simulink model "Stabilize_HIL"  (R2017b)
settings: Solver=FixedStepDiscrete  StartTime=0.0  StopTime=10.0  RelTol=1e-3
undefined symbols (not defined in the file): DEG2RAD, DiscIntNeverNeededParam, Kd_PITCH_AngleRate, Kd_ROLL_AngleRate, Kd_YAW_AngleRate, Ki_PITCH_AngleRate, Ki_ROLL_AngleRate, Ki_YAW_AngleRate, Kp_PITCH_ANGLE, Kp_PITCH_AngleRate, Kp_ROLL_ANGLE, Kp_ROLL_AngleRate, Kp_YAW_AngleRate, Kpxp, Kpyp, Kpzp, Kvxd, Kvxi, Kvxp, Kvyd, Kvyi, Kvyp, Kvzd, Kvzi, Kvzp, MAX_CONTROL_ANGLE_PITCH, MAX_CONTROL_ANGLE_RATE_PITCH, MAX_CONTROL_ANGLE_RATE_ROLL, MAX_CONTROL_ANGLE_RATE_Y, MAX_CONTROL_ANGLE_ROLL, MAX_CONTROL_VELOCITY_XY, MAX_CONTROL_VELOCITY_Z, RGBLED_COLOR_ENUM, RGBLED_MODE_ENUM, Saturation_I_ah, Saturation_I_az, Saturation_I_RP_Max, Saturation_I_RP_Min, Saturation_I_Y_Max, Saturation_I_Y_Min, THR_HOVER
libraries: simulink x7, pixhawk_slib_sensors_actuators x4, pixhawk_slib_uORB_RW x2
settings Model: Creator=wsh  LastModifiedBy=Mr Wang
settings OptimizationCC: DefaultParameterBehavior=Inlined  MaxStackSize=64
settings DebuggingCC: ParameterTunabilityLossMsg=error
settings HardwareCC: ProdBitPerPointer=32  ProdBitPerSizeT=32  ProdBitPerPtrDiffT=32  ProdLargestAtomicInteger=Long  ProdLargestAtomicFloat=Double  ProdWordSize=32  ProdHWDeviceType=ARM Compatible->ARM Cortex
settings SFSimCC: MATLABDynamicMemAlloc=off
settings RTWCC: SystemTargetFile=ert.tlc  HardwareBoard=Pixhawk PX4  TemplateMakefile=ert_default_tmf  GenerateReport=on  Toolchain=Pixhawk Toolchain  IncludeHyperlinkInReport=on  LaunchReport=on  GenerateTraceInfo=on  GenerateTraceReport=on  GenerateTraceReportSl=on  GenerateTraceReportSf=on  GenerateTraceReportEml=on
settings CodeAppCC: ForceParamTrailComments=on  IgnoreCustomStorageClasses=off  OperatorAnnotations=on  SimulinkDataObjDesc=on  SFDataObjDesc=on  MATLABFcnDesc=on  InsertBlockDesc=on  StateflowObjectComments=on  MATLABSourceComments=on
settings ERTTargetCC: MultiwordLength=2048  ERTCustomFileTemplate=PX4_codertarget_file_process.tlc

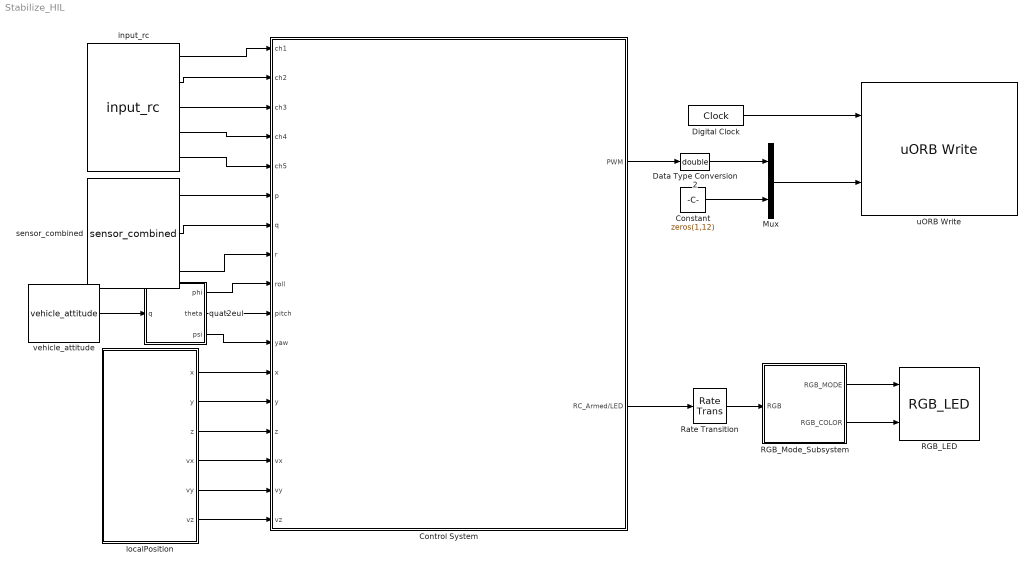
== system Stabilize_HIL ==
  Constant : Constant  Value=zeros(1,12)
  Control System : Subsystem
      mask Display: image('icon\pixhawk.png');
  Data Type Conversion2 : DataTypeConversion  OutDataTypeStr=double
  Digital Clock : DigitalClock  SampleTime=-1
  Mux : Mux  Inputs=2
  RGB_LED : pixhawk_slib_sensors_actuators/RGB_LED
      settings: SourceProductName=Pixhawk Target Blocks
  RGB_Mode_Subsystem : Subsystem
  Rate Transition : RateTransition  OutPortSampleTime=1
  input_rc : pixhawk_slib_sensors_actuators/input_rc  Description=|  sampletime=0.004  channel1=on  channel2=on  channel3=on  channel4=on  channel5=on  channel6=off  channel7=off  channel8=off  channel9=off  channel10=off  channel11=off  channel12=off  channel13=off  channel14=off  channel15=off  channel16=off  channel17=off  channel18=off  ch_count=off  rssi=off  rc_failsafe=off  rc_lost=off  rc_inputsource=off
      | RC Input Block
      | 
      | This block provides user input control to the model.
      | It uses the input_rc uORB topic.
      | 
      | The user has the ability to choose which channels are available as outputs from this block and also some optional outputs. These include 
      | Channels 1 through 18
      | double data type indicating the PWM value from the controller 
      | measured pulse widths for each of the supported channels 
      | Channel Count 
      | uint32 data type of the number of channels which are detector by the PX4 
      | RC Failsafe 
      | boolean data types indicating that the RC Tx is sending the FailSafe signal (if equipped and properly setup) 
      | explicit failsafe flag: true on TX failure or TX out of range , false otherwise. 
      | Only the true state is reliable, as there are some (PPM) receivers on the market going into failsafe without telling us explicitly. 
      | RC Input Source 
      | Enumeration data type indicating which source the RC input is from. 
      | Valid values are found in the ENUM file: RC_INPUT_SOURCE_ENUM.m 
      |           Enumeration members for class 'RC_INPUT_SOURCE_ENUM':
      |           RCINPUT_SOURCE_UNKNOWN         (0)
      |           RCINPUT_SOURCE_PX4FMU_PPM      (1)
      |           RCINPUT_SOURCE_PX4IO_PPM       (2)
      |           RCINPUT_SOURCE_PX4IO_SPEKTRUM  (3)
      |           RCINPUT_SOURCE_PX4IO_SBUS      (4)
      |           RCINPUT_SOURCE_PX4IO_ST24      (5)
      |           RCINPUT_SOURCE_MAVLINK         (6)
      |           RCINPUT_SOURCE_QURT            (7)
      |           RCINPUT_SOURCE_PX4FMU_SPEKTRUM (8)
      |           RCINPUT_SOURCE_PX4FMU_SBUS     (9)
      |           RCINPUT_SOURCE_PX4FMU_ST24     (10)
      |           RCINPUT_SOURCE_PX4FMU_SUMD     (11)
      |           RCINPUT_SOURCE_PX4FMU_DSM      (12)
      |           RCINPUT_SOURCE_PX4IO_SUMD      (13)
      | 
      | RSSI - Receive signal strength index 
      | receive signal strength indicator (RSSI): < 0: Undefined, 0: no signal, 255: full reception 
      | RC Lost Connection 
      | boolean data type indicating RC receiver connection status 
      | True, if no frame has arrived in the expected time, false otherwise. 
      | True usally means that the receiver has been disconnected, but can also indicate a radio link loss on "stupid" systems. 
      | Will remain false, if a RX with failsafe option continues to transmit frames after a link loss. 
      |   
      | Sample Model: px4demo_input_rc.slx
      settings: SourceProductName=Pixhawk Target Blocks
  "localPosition " : Subsystem
  quat2eul : MATLAB Function  TreatAsAtomicUnit=on
  sensor_combined : pixhawk_slib_sensors_actuators/sensor_combined  Description=|  sampletime=0.004  show_mag=off  show_acc=off  show_gyro=on  show_baro=off  show_ts=off
      | Sensor Combined Block
      | 
      | This block enables access to the various sensors available on the px4fmu-v2 hardware.  
      | The user can use these signals in the Simulink control model.  
      | The sample time needs to be provided in the mask dialog.  
      | Optional output ports can also be selected.  
      | Refer to the sample model: px4demo_attitude_control.slx
      | 
      | Signal definitions: 
      | Magnetometer (x,y,z) - single values – Magnetic field in NED body frame, in Gauss 
      | Accelerometer (x,y,z) - single values – Acceleration in NED body frame, in m/s^2 
      | Gyroscope (p,q,r) - single values – Angular velocity in radians per second 
      | Barometer (Altitude) - single value – Barometric pressure, already temperature compensated (millibars) 
      | RunTime (timestamp) - double value – Timestamp in microseconds since boot, from gyro 
      |   
      | The sensor_combined block needs to have the px4io service running on the PX4 hardware in order to get valid signal values.
      settings: SourceProductName=Pixhawk Target Blocks
  uORB Write : pixhawk_slib_uORB_RW/uORB Write  uORB_Topic_str='actuator_outputs'  BlockOutputCount=2  OutputBoolean_1=on  uORB_Param_Name1='timestamp'  uORB_Param_Name_DT1=double  VectorScalar_1=1  OutputBoolean_2=on  uORB_Param_Name2='output'  uORB_Param_Name_DT2=double  VectorScalar_2=16  OutputBoolean_3=off  uORB_Param_Name3='timestamp_time'  uORB_Param_Name_DT3=double  VectorScalar_3=1  OutputBoolean_4=off  uORB_Param_Name4='gyro_temp'  uORB_Param_Name_DT4=single  VectorScalar_4=3  OutputBoolean_5=off  uORB_Param_Name5='vel_ned_valid'  uORB_Param_Name_DT5=boolean  VectorScalar_5=1  Ts=-1  MsgSizeOf=0
      settings: SourceProductName=Pixhawk Target Blocks
  vehicle_attitude : pixhawk_slib_sensors_actuators/vehicle_attitude  Description=|  sampletime=0.004  show_r=off  show_p=off  show_y=off  show_q=on  show_ts=off
      | This block gives access to the running service that calculates the vehicle’s attitude.  A uORB topic (vehicle_attitude (attitude measurements)) publisher MUST be running in order for this block to provide valid signal values.  The available ones as of v1.3 are: 
      | attitude_estimator_ekf – EKF-Extended Kalman Filter for attitude estimation 
      | attitude_estimator_so3 – SO(3)-attitude estimation by using accelerometer, gyroscopes and magnetometer 
      | One of these MUST be running on the px4fmu in order for this block to return valid values.  Refer to the sample model: px4demo_attitude_control.slx. Attitude in NED (North-East-Down) body frame in SI units. 
      | Signal definitions: 
      | Roll – single value, Roll angle (rad, Tait-Bryan, NED) 
      | Pitch – single value, Pitch angle (rad, Tait-Bryan, NED) 
      | Yaw – single value, Yaw angle (rad, Tait-Bryan, NED) 
      | Quaternion (NED) – single(4) values (optional based on the uORB publisher)
      settings: SourceProductName=Pixhawk Target Blocks
  wires:
  sensor_combined/1 -> Control System/6(p)
  sensor_combined/3 -> Control System/8(r)
  sensor_combined/2 -> Control System/7(q)
  input_rc/5 -> Control System/5(ch5)
  input_rc/4 -> Control System/4(ch4)
  input_rc/3 -> Control System/3(ch3)
  input_rc/2 -> Control System/2(ch2)
  input_rc/1 -> Control System/1(ch1)
  quat2eul/3(psi) -> Control System/11(yaw)
  quat2eul/1(phi) -> Control System/9(roll)
  "localPosition "/6(vz) -> Control System/17(vz)
  "localPosition "/1(x) -> Control System/12(x)
  "localPosition "/3(z) -> Control System/14(z)
  "localPosition "/4(vx) -> Control System/15(vx)
  "localPosition "/2(y) -> Control System/13(y)
  vehicle_attitude/1 -> quat2eul/1(q)
  "localPosition "/5(vy) -> Control System/16(vy)
  quat2eul/2(theta) -> Control System/10(pitch)
  Control System/2(RC_Armed/LED) -> Rate Transition/1
  RGB_Mode_Subsystem/1(RGB_MODE) -> RGB_LED/1
  RGB_Mode_Subsystem/2(RGB_COLOR) -> RGB_LED/2
  Data Type Conversion2/1 -> Mux/1
  Control System/1(PWM) -> Data Type Conversion2/1
  Rate Transition/1 -> RGB_Mode_Subsystem/1(RGB)
  Constant/1 -> Mux/2
  Digital Clock/1 -> uORB Write/1
  Mux/1 -> uORB Write/2

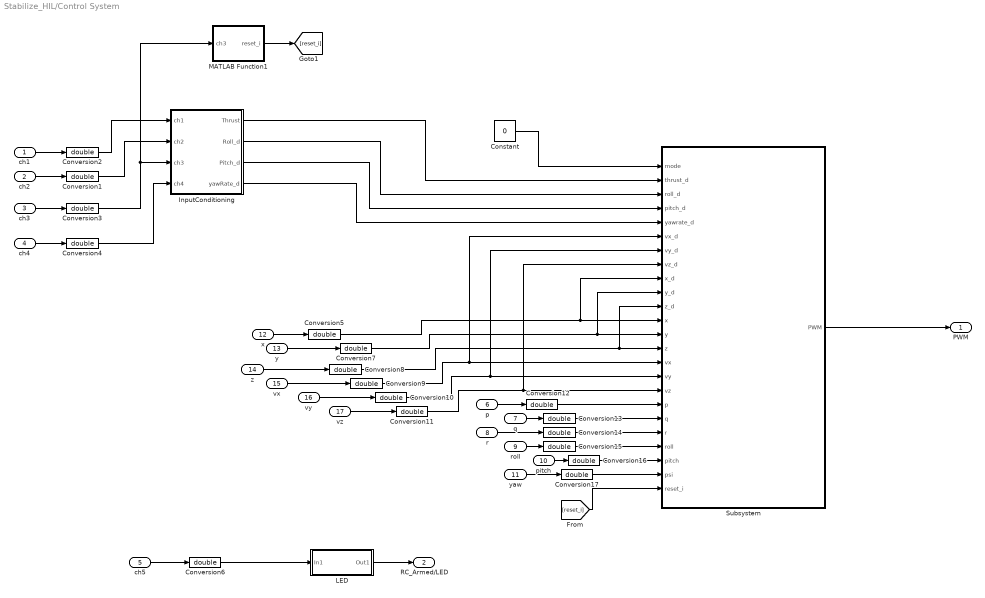
== system Stabilize_HIL/Control System ==
  ch1 : Inport  OutDataTypeStr=uint16  PortDimensions=1
  ch2 : Inport  Port=2  OutDataTypeStr=uint16  PortDimensions=1
  ch3 : Inport  Port=3  OutDataTypeStr=uint16  PortDimensions=1
  ch4 : Inport  Port=4  OutDataTypeStr=uint16  PortDimensions=1
  ch5 : Inport  Port=5  OutDataTypeStr=uint16  PortDimensions=1  Interpolate=off
  p : Inport  Port=6  PortDimensions=1
  q : Inport  Port=7  PortDimensions=1
  r : Inport  Port=8  PortDimensions=1
  roll : Inport  Port=9  PortDimensions=1
  pitch : Inport  Port=10  PortDimensions=1
  yaw : Inport  Port=11  PortDimensions=1
  x : Inport  Port=12
  y : Inport  Port=13
  z : Inport  Port=14
  vx : Inport  Port=15
  vy : Inport  Port=16
  vz : Inport  Port=17
  Constant : Constant  Value=0
  Conversion{1..17} (17 alike) : DataTypeConversion  OutDataTypeStr=double
  InputConditioning : Subsystem
  "LED " : Subsystem
  MATLAB Function1 : MATLAB Function  TreatAsAtomicUnit=on
  Subsystem : Subsystem
  PWM : Outport
  RC_Armed/LED : Outport  Port=2  PortDimensions=1
  wires:
  ch3/1 -> Conversion3/1
  ch5/1 -> Conversion6/1
  ch4/1 -> Conversion4/1
  Conversion4/1 -> InputConditioning/4(ch4)
  ch1/1 -> Conversion2/1
  ch2/1 -> Conversion1/1
  Conversion1/1 -> InputConditioning/2(ch2)
  x/1 -> Conversion5/1
  y/1 -> Conversion7/1
  z/1 -> Conversion8/1
  Constant/1 -> Subsystem/1(mode)
  roll/1 -> Conversion15/1
  pitch/1 -> Conversion16/1
  p/1 -> Conversion12/1
  q/1 -> Conversion13/1
  r/1 -> Conversion14/1
  yaw/1 -> Conversion17/1
  vz/1 -> Conversion11/1
  vy/1 -> Conversion10/1
  vx/1 -> Conversion9/1
  InputConditioning/2(Roll_d) -> Subsystem/3(roll_d)
  InputConditioning/3(Pitch_d) -> Subsystem/4(pitch_d)
  InputConditioning/1(Thrust) -> Subsystem/2(thrust_d)
  InputConditioning/4(yawRate_d) -> Subsystem/5(yawrate_d)
  Conversion5/1 -> Subsystem/12(x), Subsystem/9(x_d)
  Conversion7/1 -> Subsystem/13(y), Subsystem/10(y_d)
  Conversion8/1 -> Subsystem/14(z), Subsystem/11(z_d)
  Conversion9/1 -> Subsystem/15(vx), Subsystem/6(vx_d)
  Conversion10/1 -> Subsystem/16(vy), Subsystem/7(vy_d)
  Conversion11/1 -> Subsystem/17(vz), Subsystem/8(vz_d)
  Conversion12/1 -> Subsystem/18(p)
  Conversion13/1 -> Subsystem/19(q)
  Conversion14/1 -> Subsystem/20(r)
  Conversion15/1 -> Subsystem/21(roll)
  Conversion16/1 -> Subsystem/22(pitch)
  Conversion17/1 -> Subsystem/23(psi)
  Conversion3/1 -> MATLAB Function1/1(ch3), InputConditioning/3(ch3)
  MATLAB Function1/1(reset_i) -> [reset_i]
  [reset_i] -> Subsystem/24(reset_i)
  Conversion2/1 -> InputConditioning/1("ch1 ")
  Subsystem/1(PWM) -> PWM/1
  Conversion6/1 -> "LED "/1(In1)
  "LED "/1(Out1) -> RC_Armed/LED/1

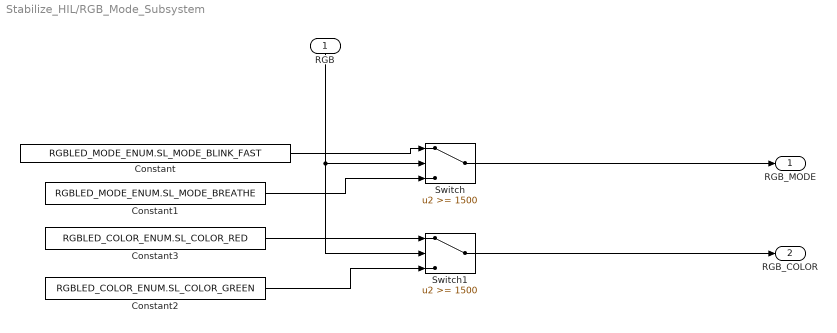
== system Stabilize_HIL/RGB_Mode_Subsystem ==
  RGB : Inport
  Constant : Constant  Value=RGBLED_MODE_ENUM.SL_MODE_BLINK_FAST  OutDataTypeStr=Enum: RGBLED_MODE_ENUM
  Constant1 : Constant  Value=RGBLED_MODE_ENUM.SL_MODE_BREATHE  OutDataTypeStr=Enum: RGBLED_MODE_ENUM
  Constant2 : Constant  Value=RGBLED_COLOR_ENUM.SL_COLOR_GREEN  OutDataTypeStr=Enum: RGBLED_COLOR_ENUM
  Constant3 : Constant  Value=RGBLED_COLOR_ENUM.SL_COLOR_RED  OutDataTypeStr=Enum: RGBLED_COLOR_ENUM
  Switch : Switch  Threshold=1500
  Switch1 : Switch  Threshold=1500
  RGB_MODE : Outport
  RGB_COLOR : Outport  Port=2
  wires:
  RGB/1 -> Switch1/2, Switch/2
  Constant/1 -> Switch/1
  Constant1/1 -> Switch/3
  Switch/1 -> RGB_MODE/1
  Constant3/1 -> Switch1/1
  Constant2/1 -> Switch1/3
  Switch1/1 -> RGB_COLOR/1

== system Stabilize_HIL/localPosition  ==
  Bus Selector2 : BusSelector  OutputSignals=x,y,z,vx,vy,vz
  uORB Read Function-Call Trigger : pixhawk_slib_uORB_RW/uORB Read Function-Call Trigger  uORB_Topic_str='vehicle_local_position'  BusObjVar=Bus: vehicle_local_position_SL  uORB_Interval=1  AsyncOutput=off  Fcn_call_select=Generate Function Call Signal  TaskName='Task1'  Poll_timeout=100  Ts=-1
      settings: SourceProductName=Pixhawk Target Blocks
  x : Outport
  y : Outport  Port=2
  z : Outport  Port=3
  vx : Outport  Port=4
  vy : Outport  Port=5
  vz : Outport  Port=6
  wires:
  uORB Read Function-Call Trigger/1 -> Bus Selector2/1
  Bus Selector2/6 -> vz/1  "<vz>"
  Bus Selector2/5 -> vy/1  "<vy>"
  Bus Selector2/4 -> vx/1  "<vx>"
  Bus Selector2/1 -> x/1  "<x>"
  Bus Selector2/2 -> y/1  "<y>"
  Bus Selector2/3 -> z/1  "<z>"

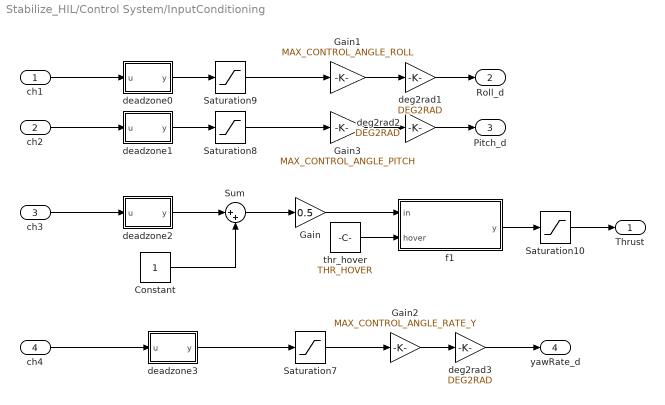
== system Stabilize_HIL/Control System/InputConditioning ==
  "ch1 " : Inport
  ch2 : Inport  Port=2
  ch3 : Inport  Port=3
  ch4 : Inport  Port=4
  Constant : Constant
  Gain : Gain  Gain=0.5
  Gain1 : Gain  Gain=MAX_CONTROL_ANGLE_ROLL  OutDataTypeStr=Inherit: Inherit via back propagation
  Gain2 : Gain  Gain=MAX_CONTROL_ANGLE_RATE_Y
  Gain3 : Gain  Gain=MAX_CONTROL_ANGLE_PITCH  OutDataTypeStr=Inherit: Inherit via back propagation
  Saturation10 : Saturate  UpperLimit=1  LowerLimit=0
  Saturation7 : Saturate  UpperLimit=1  LowerLimit=-1
  Saturation8 : Saturate  UpperLimit=1  LowerLimit=-1
  Saturation9 : Saturate  UpperLimit=1  LowerLimit=-1
  Sum : Sum  Inputs=|++
  deadzone0 : MATLAB Function  TreatAsAtomicUnit=on
  deadzone1 : MATLAB Function  TreatAsAtomicUnit=on
  deadzone2 : MATLAB Function  TreatAsAtomicUnit=on
  deadzone3 : MATLAB Function  TreatAsAtomicUnit=on
  deg2rad1 : Gain  Gain=DEG2RAD
  deg2rad2 : Gain  Gain=DEG2RAD
  deg2rad3 : Gain  Gain=DEG2RAD
  f1 : MATLAB Function  TreatAsAtomicUnit=on
  "thr_hover " : Constant  Value=THR_HOVER
  Thrust : Outport
  Roll_d : Outport  Port=2
  Pitch_d : Outport  Port=3
  yawRate_d : Outport  Port=4
  wires:
  deadzone2/1(y) -> Sum/1
  ch3/1 -> deadzone2/1(u)
  deadzone1/1(y) -> Saturation8/1
  Saturation10/1 -> Thrust/1
  deadzone0/1(y) -> Saturation9/1
  "ch1 "/1 -> deadzone0/1(u)
  ch2/1 -> deadzone1/1(u)
  Saturation9/1 -> Gain1/1
  Saturation8/1 -> Gain3/1
  Gain3/1 -> deg2rad2/1
  Constant/1 -> Sum/2
  Sum/1 -> Gain/1
  Gain1/1 -> deg2rad1/1
  deg2rad1/1 -> Roll_d/1
  deg2rad2/1 -> Pitch_d/1
  Saturation7/1 -> Gain2/1
  deadzone3/1(y) -> Saturation7/1
  ch4/1 -> deadzone3/1(u)
  Gain2/1 -> deg2rad3/1
  deg2rad3/1 -> yawRate_d/1
  "thr_hover "/1 -> f1/2(hover)
  Gain/1 -> f1/1(in)
  f1/1(y) -> Saturation10/1

== system Stabilize_HIL/Control System/LED  ==
  In1 : Inport
  Compare To Constant3 : simulink/Logic and Bit Operations/Compare To Constant  relop=>=  const=uint16(1500)  OutDataTypeStr=boolean
  Out1 : Outport
  wires:
  Compare To Constant3/1 -> Out1/1
  In1/1 -> Compare To Constant3/1

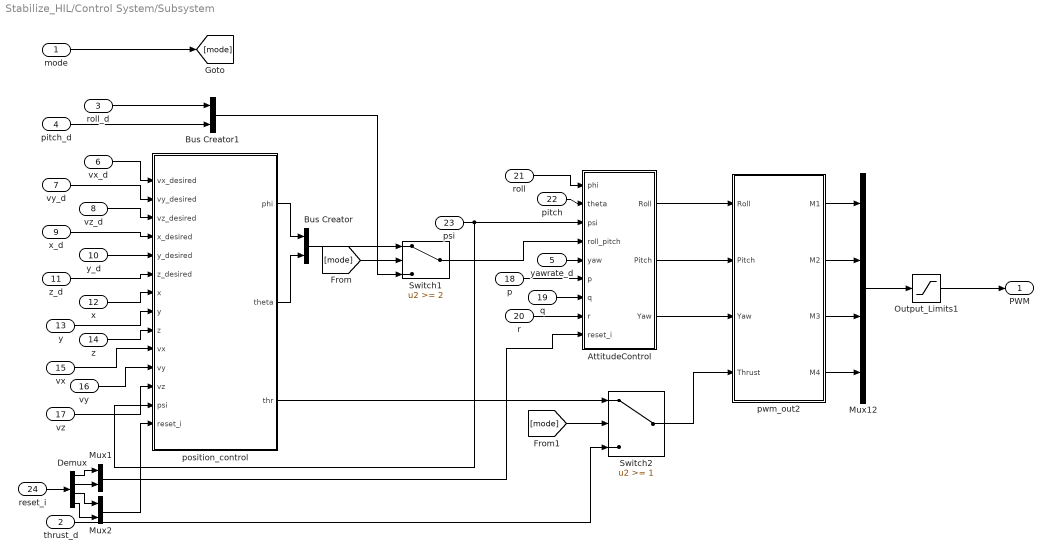
== system Stabilize_HIL/Control System/Subsystem ==
  mode : Inport
  thrust_d : Inport  Port=2
  roll_d : Inport  Port=3
  pitch_d : Inport  Port=4
  yawrate_d : Inport  Port=5
  vx_d : Inport  Port=6
  vy_d : Inport  Port=7
  vz_d : Inport  Port=8
  x_d : Inport  Port=9
  y_d : Inport  Port=10
  z_d : Inport  Port=11
  x : Inport  Port=12
  y : Inport  Port=13
  z : Inport  Port=14
  vx : Inport  Port=15
  vy : Inport  Port=16
  vz : Inport  Port=17
  p : Inport  Port=18  PortDimensions=1
  q : Inport  Port=19  PortDimensions=1
  r : Inport  Port=20  PortDimensions=1
  roll : Inport  Port=21  PortDimensions=1
  pitch : Inport  Port=22  PortDimensions=1
  psi : Inport  Port=23  PortDimensions=1
  reset_i : Inport  Port=24
  AttitudeControl : Subsystem
  Bus Creator : BusCreator  Inputs=2
  Bus Creator1 : BusCreator  Inputs=2
  Demux : Demux
  Mux1 : Mux  Inputs=2
  Mux12 : Mux
  Mux2 : Mux  Inputs=2
  Output_Limits1 : Saturate  UpperLimit=2000  LowerLimit=1000
  Switch1 : Switch  Threshold=2
  Switch2 : Switch  Threshold=1
  position_control : Subsystem
  pwm_out2 : MATLAB Function  SystemSampleTime=0.004
  PWM : Outport
  wires:
  pwm_out2/4(M4) -> Mux12/4
  pwm_out2/3(M3) -> Mux12/3
  yawrate_d/1 -> AttitudeControl/5(yaw)
  roll/1 -> AttitudeControl/1(phi)
  Output_Limits1/1 -> PWM/1
  q/1 -> AttitudeControl/7(q)
  AttitudeControl/1(Roll) -> pwm_out2/1(Roll)
  pwm_out2/2(M2) -> Mux12/2
  AttitudeControl/2(Pitch) -> pwm_out2/2(Pitch)
  pitch/1 -> AttitudeControl/2(theta)
  Mux12/1 -> Output_Limits1/1
  position_control/2(theta) -> Bus Creator/2
  pwm_out2/1(M1) -> Mux12/1
  AttitudeControl/3(Yaw) -> pwm_out2/3(Yaw)
  position_control/1(phi) -> Bus Creator/1
  p/1 -> AttitudeControl/6(p)
  vx/1 -> position_control/10(vx)
  vz/1 -> position_control/12(vz)
  vy/1 -> position_control/11(vy)
  x_d/1 -> position_control/4(x_desired)
  y_d/1 -> position_control/5(y_desired)
  z_d/1 -> position_control/6(z_desired)
  mode/1 -> [mode]
  vz_d/1 -> position_control/3(vz_desired)
  x/1 -> position_control/7(x)
  vx_d/1 -> position_control/1(vx_desired)
  vy_d/1 -> position_control/2(vy_desired)
  y/1 -> position_control/8(y)
  z/1 -> position_control/9(z)
  Bus Creator/1 -> Switch1/1
  [mode] -> Switch1/2
  Switch1/1 -> AttitudeControl/4(roll_pitch)
  roll_d/1 -> Bus Creator1/1
  pitch_d/1 -> Bus Creator1/2
  Bus Creator1/1 -> Switch1/3
  [mode] -> Switch2/2
  position_control/3(thr) -> Switch2/1
  Switch2/1 -> pwm_out2/4(Thrust)
  thrust_d/1 -> Switch2/3
  r/1 -> AttitudeControl/8(r)
  psi/1 -> AttitudeControl/3(psi), position_control/13(psi)
  reset_i/1 -> Demux/1
  Mux2/1 -> position_control/14(reset_i)
  Mux1/1 -> AttitudeControl/9(reset_i)
  Demux/1 -> Mux1/1
  Demux/2 -> Mux1/2
  Demux/3 -> Mux2/1
  Demux/4 -> Mux2/2

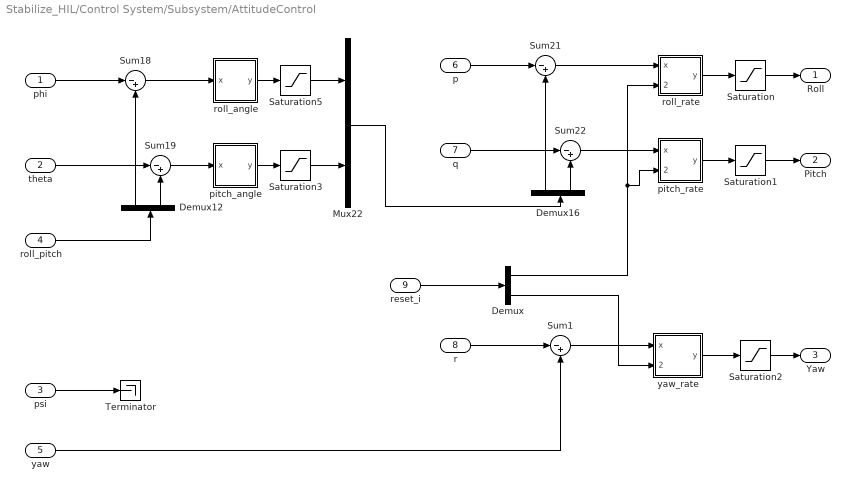
== system Stabilize_HIL/Control System/Subsystem/AttitudeControl ==
  phi : Inport
  theta : Inport  Port=2
  psi : Inport  Port=3
  roll_pitch : Inport  Port=4
  yaw : Inport  Port=5
  p : Inport  Port=6
  q : Inport  Port=7
  r : Inport  Port=8
  reset_i : Inport  Port=9
  Demux : Demux  Outputs=2
  Demux12 : Demux  Outputs=2
  Demux16 : Demux  Outputs=2
  Mux22 : Mux  Inputs=2
  Saturation : Saturate  UpperLimit=1  LowerLimit=-1
  Saturation1 : Saturate  UpperLimit=1  LowerLimit=-1
  Saturation2 : Saturate
  Saturation3 : Saturate  UpperLimit=MAX_CONTROL_ANGLE_RATE_PITCH  LowerLimit=-MAX_CONTROL_ANGLE_RATE_PITCH
  Saturation5 : Saturate  UpperLimit=MAX_CONTROL_ANGLE_RATE_ROLL  LowerLimit=-MAX_CONTROL_ANGLE_RATE_ROLL
  Sum1 : Sum  Inputs=|-+
  Sum18 : Sum  Inputs=|-+  OutMin=-90  OutMax=90
  Sum19 : Sum  Inputs=|-+  OutMin=-90  OutMax=90
  Sum21 : Sum  Inputs=|-+
  Sum22 : Sum  Inputs=|-+
  Terminator : Terminator
  "pitch_angle " : Subsystem
  pitch_rate : Subsystem
  "roll_angle " : Subsystem
  roll_rate : Subsystem
  yaw_rate : Subsystem
  Roll : Outport
  Pitch : Outport  Port=2
  Yaw : Outport  Port=3
  wires:
  Sum19/1 -> "pitch_angle "/1(x)
  "pitch_angle "/1(y) -> Saturation3/1
  Demux12/1 -> Sum18/2
  Demux12/2 -> Sum19/2
  phi/1 -> Sum18/1
  theta/1 -> Sum19/1
  Sum18/1 -> "roll_angle "/1(x)
  Sum22/1 -> pitch_rate/1(x)
  p/1 -> Sum21/1
  q/1 -> Sum22/1
  Sum21/1 -> roll_rate/1(x)
  Demux16/1 -> Sum21/2
  pitch_rate/1(y) -> Saturation1/1
  roll_rate/1(y) -> Saturation/1
  yaw_rate/1(y) -> Saturation2/1
  roll_pitch/1 -> Demux12/1
  Saturation/1 -> Roll/1
  Saturation1/1 -> Pitch/1
  Saturation2/1 -> Yaw/1
  Demux16/2 -> Sum22/2
  Mux22/1 -> Demux16/1
  r/1 -> Sum1/1
  Sum1/1 -> yaw_rate/1(x)
  "roll_angle "/1(y) -> Saturation5/1
  Saturation5/1 -> Mux22/1
  Saturation3/1 -> Mux22/2
  yaw/1 -> Sum1/2
  Demux/1 -> roll_rate/2(reset_i), pitch_rate/2(reset_i)
  reset_i/1 -> Demux/1
  Demux/2 -> yaw_rate/2(reset_i)
  psi/1 -> Terminator/1

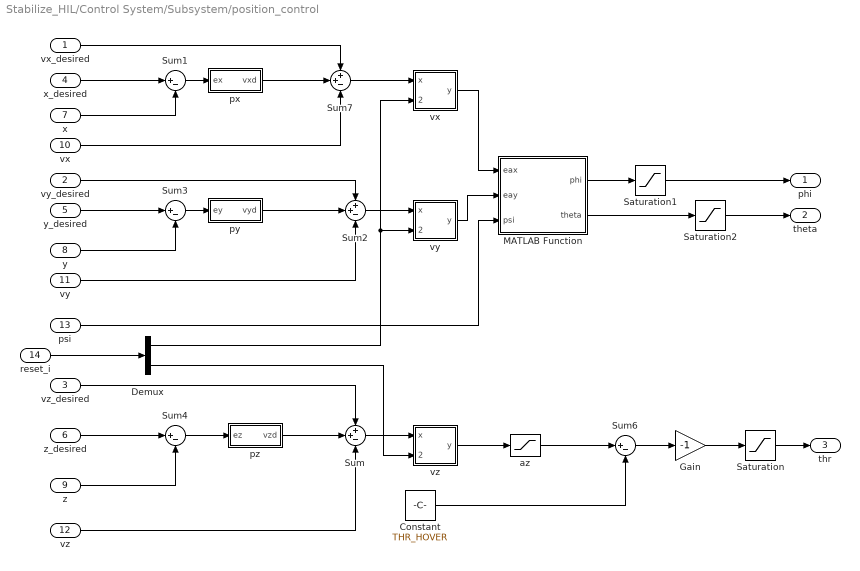
== system Stabilize_HIL/Control System/Subsystem/position_control ==
  vx_desired : Inport
  vy_desired : Inport  Port=2
  vz_desired : Inport  Port=3
  x_desired : Inport  Port=4
  y_desired : Inport  Port=5
  z_desired : Inport  Port=6
  x : Inport  Port=7
  y : Inport  Port=8
  z : Inport  Port=9
  vx : Inport  Port=10
  vy : Inport  Port=11
  vz : Inport  Port=12
  psi : Inport  Port=13
  reset_i : Inport  Port=14
  Constant : Constant  Value=THR_HOVER
  Demux : Demux  Outputs=2
  Gain : Gain  Gain=-1
  MATLAB Function : MATLAB Function  TreatAsAtomicUnit=on
  Saturation : Saturate  UpperLimit=0.9  LowerLimit=0
  Saturation1 : Saturate  UpperLimit=MAX_CONTROL_ANGLE_ROLL*DEG2RAD  LowerLimit=-MAX_CONTROL_ANGLE_ROLL*DEG2RAD
  Saturation2 : Saturate  UpperLimit=MAX_CONTROL_ANGLE_PITCH*DEG2RAD/2  LowerLimit=-MAX_CONTROL_ANGLE_PITCH*DEG2RAD/2
  Sum : Sum  Inputs=++-
  Sum{1,3..4,6} (4 alike) : Sum  Inputs=|+-
  Sum2 : Sum  Inputs=++-
  Sum7 : Sum  Inputs=++-
  az : Saturate  UpperLimit=0.4  LowerLimit=-0.4
  px : Subsystem
  py : Subsystem
  pz : Subsystem
  "vx " : Subsystem
  "vy " : Subsystem
  "vz " : Subsystem
  phi : Outport
  theta : Outport  Port=2
  thr : Outport  Port=3
  wires:
  Saturation/1 -> thr/1
  Gain/1 -> Saturation/1
  Sum6/1 -> Gain/1
  "vz "/1(y) -> az/1
  Sum4/1 -> pz/1(ez)
  z/1 -> Sum4/2
  Constant/1 -> Sum6/2
  Sum/1 -> "vz "/1(x)
  vz/1 -> Sum/3
  vx/1 -> Sum7/3
  x/1 -> Sum1/2
  y/1 -> Sum3/2
  Sum3/1 -> py/1(ey)
  y_desired/1 -> Sum3/1
  vy/1 -> Sum2/3
  Sum2/1 -> "vy "/1(x)
  Sum7/1 -> "vx "/1(x)
  Sum1/1 -> px/1(ex)
  vy_desired/1 -> Sum2/1
  py/1(vyd) -> Sum2/2
  pz/1(vzd) -> Sum/2
  z_desired/1 -> Sum4/1
  vz_desired/1 -> Sum/1
  "vx "/1(y) -> MATLAB Function/1(eax)
  px/1(vxd) -> Sum7/2
  Saturation1/1 -> phi/1
  Saturation2/1 -> theta/1
  x_desired/1 -> Sum1/1
  vx_desired/1 -> Sum7/1
  "vy "/1(y) -> MATLAB Function/2(eay)
  psi/1 -> MATLAB Function/3(psi)
  MATLAB Function/1(phi) -> Saturation1/1
  MATLAB Function/2(theta) -> Saturation2/1
  reset_i/1 -> Demux/1
  Demux/1 -> "vy "/2(reset_i), "vx "/2(reset_i)
  Demux/2 -> "vz "/2(reset_i)
  az/1 -> Sum6/1

== system Stabilize_HIL/Control System/Subsystem/AttitudeControl/pitch_angle  ==
  x : Inport
  Gain : Gain  Gain=Kp_PITCH_ANGLE
  y : Outport  InitialOutput=0
  wires:
  x/1 -> Gain/1
  Gain/1 -> y/1

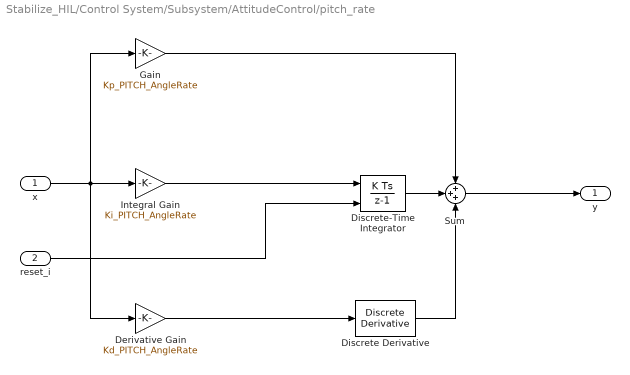
== system Stabilize_HIL/Control System/Subsystem/AttitudeControl/pitch_rate ==
  x : Inport
  reset_i : Inport  Port=2
  Derivative Gain : Gain  DisableCoverage=on  Gain=Kd_PITCH_AngleRate  ParamMin=-100  ParamMax=100  OutMin=-100  OutMax=100
  Discrete Derivative : simulink/Discrete/Discrete Derivative  gainval=1.0  ICPrevScaledInput=0.0  OutMin=[]  OutMax=[]  OutDataType=fixdt(1, 16)  OutScaling=2^-10  DoSatur=off
  Discrete-Time Integrator : DiscreteIntegrator  ExternalReset=level  InitialConditionSetting=State (most efficient)  SampleTime=-1  LimitOutput=on  UpperSaturationLimit=Saturation_I_RP_Max  LowerSaturationLimit=Saturation_I_RP_Min  ICPrevOutput=DiscIntNeverNeededParam  ICPrevScaledInput=DiscIntNeverNeededParam
  Gain : Gain  Gain=Kp_PITCH_AngleRate
  Integral Gain : Gain  DisableCoverage=on  Gain=Ki_PITCH_AngleRate
  Sum : Sum  Inputs=+++
  y : Outport  InitialOutput=0
  wires:
  Discrete-Time Integrator/1 -> Sum/2
  Discrete Derivative/1 -> Sum/3
  Sum/1 -> y/1
  Gain/1 -> Sum/1
  Derivative Gain/1 -> Discrete Derivative/1
  Integral Gain/1 -> Discrete-Time Integrator/1
  x/1 -> Derivative Gain/1, Integral Gain/1, Gain/1
  reset_i/1 -> Discrete-Time Integrator/2

== system Stabilize_HIL/Control System/Subsystem/AttitudeControl/roll_angle  ==
  x : Inport
  Gain : Gain  Gain=Kp_ROLL_ANGLE
  y : Outport  InitialOutput=0
  wires:
  Gain/1 -> y/1
  x/1 -> Gain/1

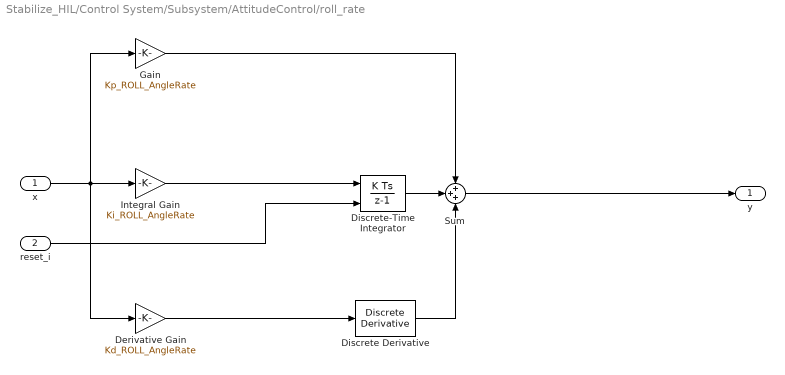
== system Stabilize_HIL/Control System/Subsystem/AttitudeControl/roll_rate ==
  x : Inport
  reset_i : Inport  Port=2
  Derivative Gain : Gain  DisableCoverage=on  Gain=Kd_ROLL_AngleRate  ParamMin=-100  ParamMax=100  OutMin=-100  OutMax=100
  Discrete Derivative : simulink/Discrete/Discrete Derivative  gainval=1.0  ICPrevScaledInput=0.0  OutMin=[]  OutMax=[]  OutDataType=fixdt(1, 16)  OutScaling=2^-10  DoSatur=off
  Discrete-Time Integrator : DiscreteIntegrator  ExternalReset=level  InitialConditionSetting=State (most efficient)  SampleTime=-1  LimitOutput=on  UpperSaturationLimit=Saturation_I_RP_Max  LowerSaturationLimit=Saturation_I_RP_Min  ICPrevOutput=DiscIntNeverNeededParam  ICPrevScaledInput=DiscIntNeverNeededParam
  Gain : Gain  Gain=Kp_ROLL_AngleRate
  Integral Gain : Gain  DisableCoverage=on  Gain=Ki_ROLL_AngleRate
  Sum : Sum  Inputs=+++
  y : Outport  InitialOutput=0
  wires:
  x/1 -> Gain/1, Integral Gain/1, Derivative Gain/1
  Integral Gain/1 -> Discrete-Time Integrator/1
  Derivative Gain/1 -> Discrete Derivative/1
  Gain/1 -> Sum/1
  Sum/1 -> y/1
  Discrete Derivative/1 -> Sum/3
  Discrete-Time Integrator/1 -> Sum/2
  reset_i/1 -> Discrete-Time Integrator/2

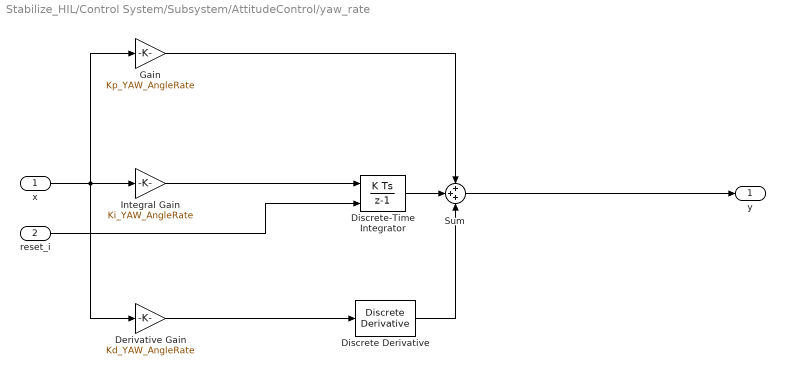
== system Stabilize_HIL/Control System/Subsystem/AttitudeControl/yaw_rate ==
  x : Inport
  reset_i : Inport  Port=2
  Derivative Gain : Gain  DisableCoverage=on  Gain=Kd_YAW_AngleRate  ParamMin=-100  ParamMax=100  OutMin=-100  OutMax=100
  Discrete Derivative : simulink/Discrete/Discrete Derivative  gainval=1.0  ICPrevScaledInput=0.0  OutMin=[]  OutMax=[]  OutDataType=fixdt(1, 16)  OutScaling=2^-10  DoSatur=off
  Discrete-Time Integrator : DiscreteIntegrator  ExternalReset=level  InitialConditionSetting=State (most efficient)  SampleTime=-1  LimitOutput=on  UpperSaturationLimit=Saturation_I_Y_Max  LowerSaturationLimit=Saturation_I_Y_Min  ICPrevOutput=DiscIntNeverNeededParam  ICPrevScaledInput=DiscIntNeverNeededParam
  Gain : Gain  Gain=Kp_YAW_AngleRate
  Integral Gain : Gain  DisableCoverage=on  Gain=Ki_YAW_AngleRate
  Sum : Sum  Inputs=+++
  y : Outport  InitialOutput=0
  wires:
  x/1 -> Gain/1, Integral Gain/1, Derivative Gain/1
  Integral Gain/1 -> Discrete-Time Integrator/1
  Derivative Gain/1 -> Discrete Derivative/1
  Gain/1 -> Sum/1
  Sum/1 -> y/1
  Discrete Derivative/1 -> Sum/3
  Discrete-Time Integrator/1 -> Sum/2
  reset_i/1 -> Discrete-Time Integrator/2

== system Stabilize_HIL/Control System/Subsystem/position_control/px ==
  ex : Inport
  Gain1 : Gain  Gain=Kpxp
  Saturation3 : Saturate  UpperLimit=MAX_CONTROL_VELOCITY_XY  LowerLimit=-MAX_CONTROL_VELOCITY_XY
  vxd : Outport
  wires:
  ex/1 -> Gain1/1
  Saturation3/1 -> vxd/1
  Gain1/1 -> Saturation3/1

== system Stabilize_HIL/Control System/Subsystem/position_control/py ==
  ey : Inport
  Gain1 : Gain  Gain=Kpyp
  Saturation3 : Saturate  UpperLimit=MAX_CONTROL_VELOCITY_XY  LowerLimit=-MAX_CONTROL_VELOCITY_XY
  vyd : Outport
  wires:
  Gain1/1 -> Saturation3/1
  Saturation3/1 -> vyd/1
  ey/1 -> Gain1/1

== system Stabilize_HIL/Control System/Subsystem/position_control/pz ==
  ez : Inport
  Gain1 : Gain  Gain=Kpzp
  Saturation3 : Saturate  UpperLimit=MAX_CONTROL_VELOCITY_Z  LowerLimit=-MAX_CONTROL_VELOCITY_Z
  vzd : Outport
  wires:
  ez/1 -> Gain1/1
  Saturation3/1 -> vzd/1
  Gain1/1 -> Saturation3/1

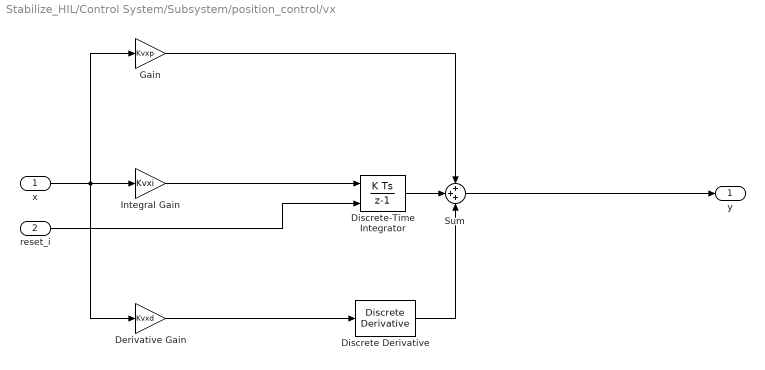
== system Stabilize_HIL/Control System/Subsystem/position_control/vx  ==
  x : Inport
  reset_i : Inport  Port=2
  Derivative Gain : Gain  DisableCoverage=on  Gain=Kvxd
  Discrete Derivative : simulink/Discrete/Discrete Derivative  gainval=1.0  ICPrevScaledInput=0.0  OutMin=[]  OutMax=[]  OutDataType=fixdt(1, 16)  OutScaling=2^-10  DoSatur=off
  Discrete-Time Integrator : DiscreteIntegrator  ExternalReset=level  InitialConditionSetting=State (most efficient)  SampleTime=-1  LimitOutput=on  UpperSaturationLimit=Saturation_I_ah  LowerSaturationLimit=-Saturation_I_ah  ICPrevOutput=DiscIntNeverNeededParam  ICPrevScaledInput=DiscIntNeverNeededParam
  Gain : Gain  Gain=Kvxp
  Integral Gain : Gain  DisableCoverage=on  Gain=Kvxi
  Sum : Sum  Inputs=+++
  y : Outport  InitialOutput=0
  wires:
  x/1 -> Gain/1, Integral Gain/1, Derivative Gain/1
  Integral Gain/1 -> Discrete-Time Integrator/1
  Derivative Gain/1 -> Discrete Derivative/1
  Gain/1 -> Sum/1
  Sum/1 -> y/1
  Discrete Derivative/1 -> Sum/3
  Discrete-Time Integrator/1 -> Sum/2
  reset_i/1 -> Discrete-Time Integrator/2

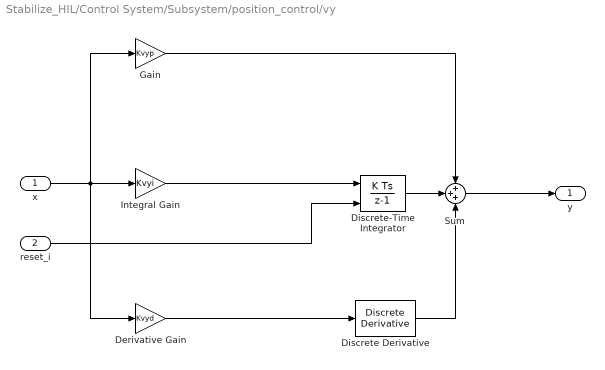
== system Stabilize_HIL/Control System/Subsystem/position_control/vy  ==
  x : Inport
  reset_i : Inport  Port=2
  Derivative Gain : Gain  DisableCoverage=on  Gain=Kvyd
  Discrete Derivative : simulink/Discrete/Discrete Derivative  gainval=1.0  ICPrevScaledInput=0.0  OutMin=[]  OutMax=[]  OutDataType=fixdt(1, 16)  OutScaling=2^-10  DoSatur=off
  Discrete-Time Integrator : DiscreteIntegrator  ExternalReset=level  InitialConditionSetting=State (most efficient)  SampleTime=-1  LimitOutput=on  UpperSaturationLimit=Saturation_I_ah  LowerSaturationLimit=-Saturation_I_ah  ICPrevOutput=DiscIntNeverNeededParam  ICPrevScaledInput=DiscIntNeverNeededParam
  Gain : Gain  Gain=Kvyp
  Integral Gain : Gain  DisableCoverage=on  Gain=Kvyi
  Sum : Sum  Inputs=+++
  y : Outport  InitialOutput=0
  wires:
  x/1 -> Gain/1, Integral Gain/1, Derivative Gain/1
  Integral Gain/1 -> Discrete-Time Integrator/1
  Derivative Gain/1 -> Discrete Derivative/1
  Gain/1 -> Sum/1
  Sum/1 -> y/1
  Discrete Derivative/1 -> Sum/3
  Discrete-Time Integrator/1 -> Sum/2
  reset_i/1 -> Discrete-Time Integrator/2

== system Stabilize_HIL/Control System/Subsystem/position_control/vz  ==
  x : Inport
  reset_i : Inport  Port=2
  Derivative Gain : Gain  DisableCoverage=on  Gain=Kvzd
  Discrete Derivative : simulink/Discrete/Discrete Derivative  gainval=1.0  ICPrevScaledInput=0.0  OutMin=[]  OutMax=[]  OutDataType=fixdt(1, 16)  OutScaling=2^-10  DoSatur=off
  Discrete-Time Integrator : DiscreteIntegrator  ExternalReset=level  InitialConditionSetting=State (most efficient)  SampleTime=-1  LimitOutput=on  UpperSaturationLimit=Saturation_I_az  LowerSaturationLimit=-Saturation_I_az  ICPrevOutput=DiscIntNeverNeededParam  ICPrevScaledInput=DiscIntNeverNeededParam
  Gain : Gain  Gain=Kvzp
  Integral Gain : Gain  DisableCoverage=on  Gain=Kvzi
  Sum : Sum  Inputs=+++
  y : Outport  InitialOutput=0
  wires:
  Discrete-Time Integrator/1 -> Sum/2
  Discrete Derivative/1 -> Sum/3
  Sum/1 -> y/1
  Gain/1 -> Sum/1
  Derivative Gain/1 -> Discrete Derivative/1
  Integral Gain/1 -> Discrete-Time Integrator/1
  x/1 -> Derivative Gain/1, Integral Gain/1, Gain/1
  reset_i/1 -> Discrete-Time Integrator/2

== matlab function Stabilize_HIL/Control System/MATLAB Function1 ==
  data: reset_i output; ch3 input
function reset_i= fcn(ch3)
%Function description:
%  Reset Integral when throttle < 1250
if ch3<1250
    reset_i=[1 1 1 1];
else
    reset_i=[0 0 0 0];
end

== matlab function Stabilize_HIL/quat2eul ==
  data: q input; phi output; theta output; psi output
function [phi,theta,psi] = quat2eul(q)
% Conversion from Quaternion to Euler angles based on the PX4 Firmware
% v1.6.5 release.
% 
% Quaternion -> DCM -> Euler Angles
% INPUT:
%   q: Quaternion vector of the format: (a + bi + cj + dk)
% OUTPUT:
%   [phi,theta,psi]: Euler angles in radians.
% 
 
    a = q(1);
    b = q(2);
    c = q(3);
    d = q(4);

    aSq = a*a;
    bSq = b*b;
    cSq = c*c;
    dSq = d*d;

    d_pi2 = pi/2;

    % quaternion_to_dcm
    dcm00 = aSq + bSq - cSq - dSq;
    % dcm01 = 2*(b*c - a*d);
    dcm02 = 2*(a*c + b*d);
    dcm10 = 2*(b*c + a*d);
    % dcm11 = aSq - bSq + cSq - dSq;
    dcm12 = 2*(c*d - a*b);
    dcm20 = 2*(b*d - a*c);
    dcm21 = 2*(a*b + c*d);
    dcm22 = aSq - bSq - cSq + dSq;

    % dcm_to_euler
    theta = asin(-dcm20);
    if abs(theta - d_pi2) < 1.0e-3
        phi = single(0.0);
        psi = atan2(dcm12, dcm02);
    elseif abs(theta + d_pi2) < 1.0e-3
        phi = single(0.0);
        psi = atan2(-dcm12, -dcm02);
    else
        phi = atan2(dcm21, dcm22);
        psi = atan2(dcm10, dcm00);
    end

end

== matlab function Stabilize_HIL/Control System/Subsystem/position_control/MATLAB Function ==
  data: eax input; eay input; psi input; phi output; theta output
function [phi, theta] = fcn(eax, eay, psi)
%Function description:
%  Convert the desired horizontal acceleration to the desired attitude angle
%Input:
%  eax, eaxy: desired horizontal acceleration
%  psi: yaw
%Output:
%  phi, theta: desired roll angle and desired pitch angle
g = 9.8;
phi = (-sin(psi)*eax + cos(psi)*eay)/g;
theta = (-cos(psi)*eax - sin(psi)*eay)/g;

== matlab function Stabilize_HIL/Control System/InputConditioning/deadzone0 ==
  data: u input; y output
function y = fcn(u)
%Function description:
%  Control the range of the remote control input from RCMin to RCMax, and set
%  a dead zone with a dead zone size of ±deadZone,the output y is
%  normalized to 0~1.You can get the RC calibration parameters in QGC.
RCMin = 1100;
RCMax = 1900;
RCMid = (RCMin + RCMax)/2;
deadZoneRate = 0.05;
deadZone = deadZoneRate*(RCMax - RCMin);
k = 1/(RCMax - RCMid - deadZone);
%Limiting
if(u < RCMin)
    u = RCMin;
elseif(u > RCMax)
    u = RCMax;
end
%dead zone and normalize
 if(u > RCMid + deadZone)
    y = (u-RCMid - deadZone)*k;
 elseif(u < RCMid - deadZone)
     y = (u - RCMid + deadZone)*k;
 else
     y = 0;
 end

 end

== matlab function Stabilize_HIL/Control System/InputConditioning/deadzone1 ==
  data: u input; y output
function y = fcn(u)
%Function description:
%  Control the range of the remote control input from RCMin to RCMax, and set
%  a dead zone with a dead zone size of ±deadZone,the output y is
%  normalized to 0~1.You can get the RC calibration parameters in QGC.
RCMin = 1100;
RCMax = 1900;
RCMid = (RCMin + RCMax)/2;
deadZoneRate = 0.05;
deadZone = deadZoneRate*(RCMax - RCMin);
k = 1/(RCMax - RCMid - deadZone);
%Limiting
if(u < RCMin)
    u = RCMin;
elseif(u > RCMax)
    u = RCMax;
end
%dead zone and normalize
 if(u > RCMid + deadZone)
    y = (u-RCMid - deadZone)*k;
 elseif(u < RCMid - deadZone)
     y = (u - RCMid + deadZone)*k;
 else
     y = 0;
 end

 end

== matlab function Stabilize_HIL/Control System/InputConditioning/deadzone2 ==
  data: u input; y output
function y = fcn(u)
%Function description:
%  Control the range of the remote control input from RCMin to RCMax, and set
%  a dead zone with a dead zone size of ±deadZone,the output y is
%  normalized to 0~1.You can get the RC calibration parameters in QGC.
RCMin = 1100;
RCMax = 1900;
RCMid = (RCMin + RCMax)/2;
deadZoneRate = 0.05;
deadZone = deadZoneRate*(RCMax - RCMin);
k = 1/(RCMax - RCMid - deadZone);
%Limiting
if(u < RCMin)
    u = RCMin;
elseif(u > RCMax)
    u = RCMax;
end
%dead zone and normalize
 if(u > RCMid + deadZone)
    y = (u-RCMid - deadZone)*k;
 elseif(u < RCMid - deadZone)
     y = (u - RCMid + deadZone)*k;
 else
     y = 0;
 end

 end

== matlab function Stabilize_HIL/Control System/InputConditioning/deadzone3 ==
  data: u input; y output
function y = fcn(u)
%Function description:
%  Control the range of the remote control input from RCMin to RCMax, and set
%  a dead zone with a dead zone size of ±deadZone,the output y is
%  normalized to 0~1.You can get the RC calibration parameters in QGC.
RCMin = 1100;
RCMax = 1900;
RCMid = (RCMin + RCMax)/2;
deadZoneRate = 0.05;
deadZone = deadZoneRate*(RCMax - RCMin);
k = 1/(RCMax - RCMid - deadZone);
%Limiting
if(u < RCMin)
    u = RCMin;
elseif(u > RCMax)
    u = RCMax;
end
%dead zone and normalize
 if(u > RCMid + deadZone)
    y = (u-RCMid - deadZone)*k;
 elseif(u < RCMid - deadZone)
     y = (u - RCMid + deadZone)*k;
 else
     y = 0;
 end

 end

== matlab function Stabilize_HIL/Control System/Subsystem/pwm_out2 ==
  data: Roll input; M1 output; Pitch input; Yaw input; Thrust input; M2 output; M3 output; M4 output
function [M1, M2, M3, M4] = motor_mixer(Roll, Pitch, Yaw, Thrust)
%Function description;
%  Assign the attitude controller output to the motor control. The multi-rotor type is quadrotor-X type,
%  and the propeller serial number is as follows:
%3     1
%  \ /
%  / \
%2     4
%Input：
%  Roll, Pitch, Yaw: Attitude controller output.
%  Thrust

idle_PWM = 1000;
scale = 1000;

M1 = (Thrust - Roll + Pitch + Yaw) * scale + idle_PWM;
M2 = (Thrust + Roll - Pitch + Yaw) * scale + idle_PWM;
M3 = (Thrust + Roll + Pitch - Yaw) * scale + idle_PWM;
M4 = (Thrust - Roll - Pitch - Yaw) * scale + idle_PWM;

== matlab function Stabilize_HIL/Control System/InputConditioning/f1 ==
  data: in input; y output; hover input
function y = thr_curve(in, hover)
%Function description:
%  After this function, when the throttle is in the middle position, the output is hovering throttle hover
%Input:
%  in: Throttle normalized value, range (0~1)
%  hover: Hovering throttle value
%Output:
%  Processed throttle value
if in < 0.5
	y=2 * in * hover;
else
	y=hover + 2 * (in - 0.5) * (1.0 - hover);
end
